simulink model "INELFE_LIN"  (R2023b)
settings: Solver=ode45  StartTime=0.0  StopTime=Tsim_lin  RelTol=1e-3
undefined symbols (not defined in the file): delta_u, sim_config, ss_sys, tstep_lin
settings Model: Creator=dionm  LastModifiedBy=dionm

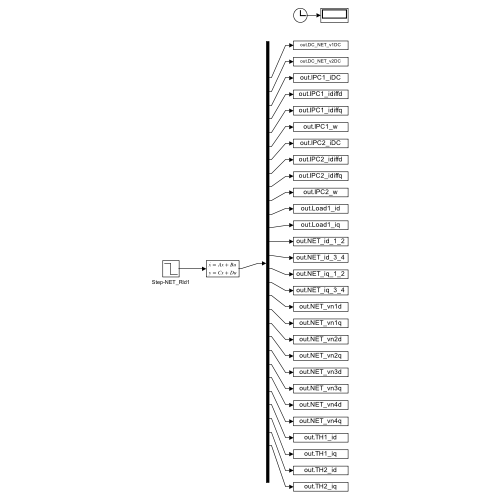
[thumbnail: Simulink's stored preview of the top-level diagram]
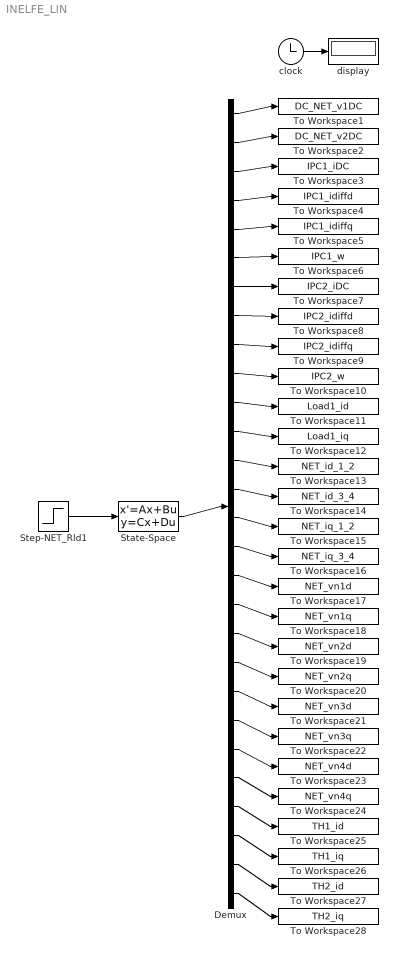
== system INELFE_LIN ==
  Demux : Demux  Outputs=28
  State-Space : StateSpace  A=ss_sys.A  B=ss_sys.B  C=ss_sys.C  D=ss_sys.D  InitialCondition=0
  Step-NET_Rld1 : Step  Time=tstep_lin  After=delta_u  SampleTime=0
  To Workspace1 : ToWorkspace  VariableName=DC_NET_v1DC  SampleTime=sim_config.Tsample
  To Workspace10 : ToWorkspace  VariableName=IPC2_w  SampleTime=sim_config.Tsample
  To Workspace11 : ToWorkspace  VariableName=Load1_id  SampleTime=sim_config.Tsample
  To Workspace12 : ToWorkspace  VariableName=Load1_iq  SampleTime=sim_config.Tsample
  To Workspace13 : ToWorkspace  VariableName=NET_id_1_2  SampleTime=sim_config.Tsample
  To Workspace14 : ToWorkspace  VariableName=NET_id_3_4  SampleTime=sim_config.Tsample
  To Workspace15 : ToWorkspace  VariableName=NET_iq_1_2  SampleTime=sim_config.Tsample
  To Workspace16 : ToWorkspace  VariableName=NET_iq_3_4  SampleTime=sim_config.Tsample
  To Workspace17 : ToWorkspace  VariableName=NET_vn1d  SampleTime=sim_config.Tsample
  To Workspace18 : ToWorkspace  VariableName=NET_vn1q  SampleTime=sim_config.Tsample
  To Workspace19 : ToWorkspace  VariableName=NET_vn2d  SampleTime=sim_config.Tsample
  To Workspace2 : ToWorkspace  VariableName=DC_NET_v2DC  SampleTime=sim_config.Tsample
  To Workspace20 : ToWorkspace  VariableName=NET_vn2q  SampleTime=sim_config.Tsample
  To Workspace21 : ToWorkspace  VariableName=NET_vn3d  SampleTime=sim_config.Tsample
  To Workspace22 : ToWorkspace  VariableName=NET_vn3q  SampleTime=sim_config.Tsample
  To Workspace23 : ToWorkspace  VariableName=NET_vn4d  SampleTime=sim_config.Tsample
  To Workspace24 : ToWorkspace  VariableName=NET_vn4q  SampleTime=sim_config.Tsample
  To Workspace25 : ToWorkspace  VariableName=TH1_id  SampleTime=sim_config.Tsample
  To Workspace26 : ToWorkspace  VariableName=TH1_iq  SampleTime=sim_config.Tsample
  To Workspace27 : ToWorkspace  VariableName=TH2_id  SampleTime=sim_config.Tsample
  To Workspace28 : ToWorkspace  VariableName=TH2_iq  SampleTime=sim_config.Tsample
  To Workspace3 : ToWorkspace  VariableName=IPC1_iDC  SampleTime=sim_config.Tsample
  To Workspace4 : ToWorkspace  VariableName=IPC1_idiffd  SampleTime=sim_config.Tsample
  To Workspace5 : ToWorkspace  VariableName=IPC1_idiffq  SampleTime=sim_config.Tsample
  To Workspace6 : ToWorkspace  VariableName=IPC1_w  SampleTime=sim_config.Tsample
  To Workspace7 : ToWorkspace  VariableName=IPC2_iDC  SampleTime=sim_config.Tsample
  To Workspace8 : ToWorkspace  VariableName=IPC2_idiffd  SampleTime=sim_config.Tsample
  To Workspace9 : ToWorkspace  VariableName=IPC2_idiffq  SampleTime=sim_config.Tsample
  clock : Clock
  display : Display
  wires:
  clock/1 -> display/1
  Step-NET_Rld1/1 -> State-Space/1
  State-Space/1 -> Demux/1
  Demux/1 -> To Workspace1/1
  Demux/2 -> To Workspace2/1
  Demux/3 -> To Workspace3/1
  Demux/4 -> To Workspace4/1
  Demux/5 -> To Workspace5/1
  Demux/6 -> To Workspace6/1
  Demux/7 -> To Workspace7/1
  Demux/8 -> To Workspace8/1
  Demux/9 -> To Workspace9/1
  Demux/10 -> To Workspace10/1
  Demux/11 -> To Workspace11/1
  Demux/12 -> To Workspace12/1
  Demux/13 -> To Workspace13/1
  Demux/14 -> To Workspace14/1
  Demux/15 -> To Workspace15/1
  Demux/16 -> To Workspace16/1
  Demux/17 -> To Workspace17/1
  Demux/18 -> To Workspace18/1
  Demux/19 -> To Workspace19/1
  Demux/20 -> To Workspace20/1
  Demux/21 -> To Workspace21/1
  Demux/22 -> To Workspace22/1
  Demux/23 -> To Workspace23/1
  Demux/24 -> To Workspace24/1
  Demux/25 -> To Workspace25/1
  Demux/26 -> To Workspace26/1
  Demux/27 -> To Workspace27/1
  Demux/28 -> To Workspace28/1
